simulink model "pid_simulation"  (R2014b)
settings: Solver=ode45  StartTime=0.0  StopTime=20  RelTol=1e-3
values from neighbouring files (symbols this model uses):
  con_D = 0    [main.m]
  con_I = 0    [main.m]
  con_P = 30    [main.m]
  k_velocity_feedback = 3.2    [main.m]
  state_initial = [0 0 0 0 0 0 0 0 0 0 0 0]    [main.m]
libraries: simulink x4
settings Model: Creator=shuoli  LastModifiedBy=shuoli

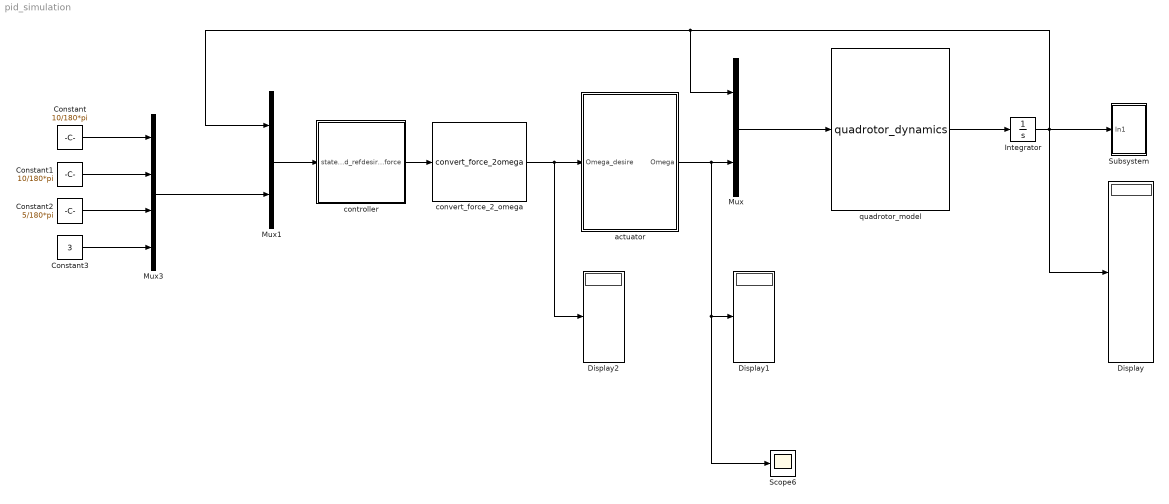
== system pid_simulation ==
  Constant : Constant  Value=10/180*pi
  Constant1 : Constant  Value=10/180*pi
  Constant2 : Constant  Value=5/180*pi
  Constant3 : Constant  Value=3
  Display : Display
  Display1 : Display
  Display2 : Display
  Integrator : Integrator  InitialCondition=state_initial
  Mux : Mux  Inputs=2
  Mux1 : Mux  Inputs=2
  Mux3 : Mux
  Scope6 : Scope
      settings: YMax=2  SaveName=ScopeData17
  Subsystem : Subsystem
  actuator : Subsystem
  controller : Subsystem
  convert_force_2_omega : MATLABFcn  MATLABFcn=convert_force_2omega
  quadrotor_model : MATLABFcn  MATLABFcn=quadrotor_dynamics
  wires:
  quadrotor_model/1 -> Integrator/1
  Mux/1 -> quadrotor_model/1
  Integrator/1 -> Display/1, Mux1/1, Mux/1, Subsystem/1(In1)
  actuator/1(Omega) -> Scope6/1, Display1/1, Mux/2
  Constant3/1 -> Mux3/4
  Constant2/1 -> Mux3/3
  Constant1/1 -> Mux3/2
  Constant/1 -> Mux3/1
  convert_force_2_omega/1 -> Display2/1, actuator/1(Omega_desire)
  Mux3/1 -> Mux1/2
  controller/1(desired_force) -> convert_force_2_omega/1
  Mux1/1 -> controller/1(state_and_ref)

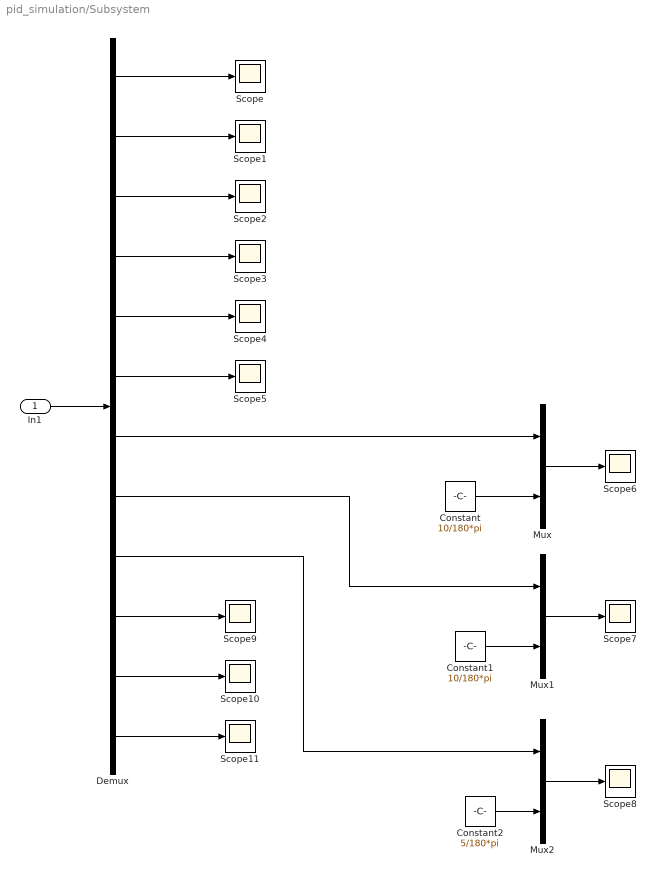
== system pid_simulation/Subsystem ==
  In1 : Inport
  Constant : Constant  Value=10/180*pi
  Constant1 : Constant  Value=10/180*pi
  Constant2 : Constant  Value=5/180*pi
  Demux : Demux  Outputs=12
  Mux : Mux  Inputs=2
  Mux1 : Mux  Inputs=2
  Mux2 : Mux  Inputs=2
  Scope{,1..11} (12 alike) : Scope
      Scope settings: YMin=186  YMax=190
      Scope10 settings: SaveName=ScopeData10
      Scope11 settings: SaveName=ScopeData11
      Scope2 settings: YMin=-18500  YMax=-16500  SaveName=ScopeData2
      Scope3 settings: SaveName=ScopeData3
      Scope4 settings: SaveName=ScopeData4
      Scope5 settings: SaveName=ScopeData5
      Scope6 settings: YMax=2  SaveName=ScopeData6
      Scope7 settings: YMax=2  SaveName=ScopeData7
      Scope8 settings: YMax=2  SaveName=ScopeData8
      Scope9 settings: SaveName=ScopeData9
  wires:
  Demux/1 -> Scope/1
  In1/1 -> Demux/1
  Demux/4 -> Scope3/1
  Demux/2 -> Scope1/1
  Demux/3 -> Scope2/1
  Demux/5 -> Scope4/1
  Demux/6 -> Scope5/1
  Demux/8 -> Mux1/1
  Demux/9 -> Mux2/1
  Demux/10 -> Scope9/1
  Demux/11 -> Scope10/1
  Demux/12 -> Scope11/1
  Demux/7 -> Mux/1
  Mux/1 -> Scope6/1
  Constant/1 -> Mux/2
  Constant1/1 -> Mux1/2
  Mux1/1 -> Scope7/1
  Constant2/1 -> Mux2/2
  Mux2/1 -> Scope8/1

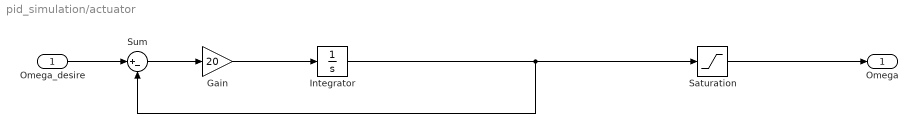
== system pid_simulation/actuator ==
  Omega_desire : Inport
  Gain : Gain  Gain=20
  Integrator : Integrator  InitialCondition=[4477,4477,4477,4477]
  Saturation : Saturate  UpperLimit=8000  LowerLimit=0
  Sum : Sum  Inputs=|+-
  Omega : Outport
  wires:
  Integrator/1 -> Sum/2, Saturation/1
  Omega_desire/1 -> Sum/1
  Sum/1 -> Gain/1
  Gain/1 -> Integrator/1
  Saturation/1 -> Omega/1

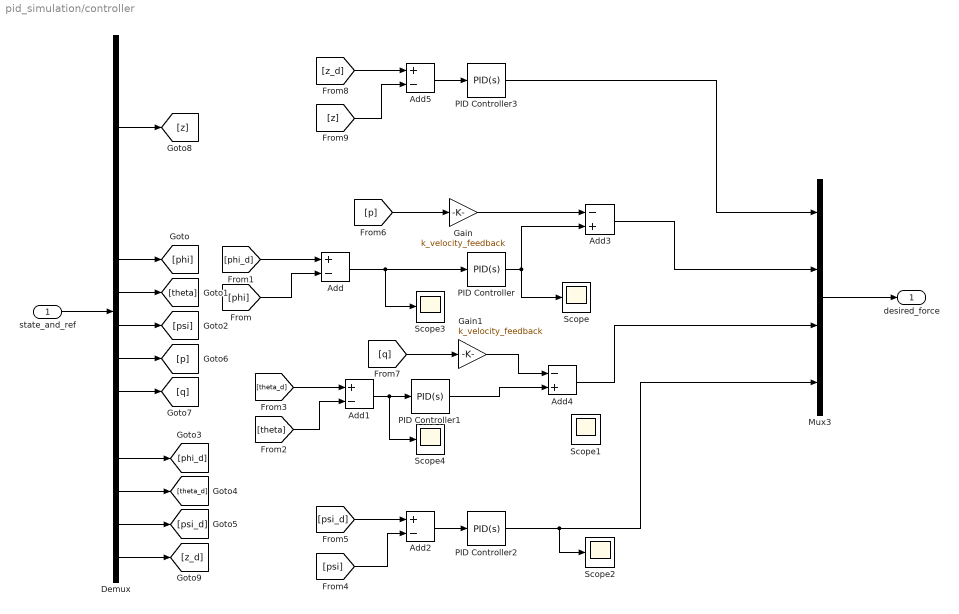
== system pid_simulation/controller ==
  state_and_ref : Inport
  Add{,1..2,5} (4 alike) : Sum  Inputs=+-
  Add3 : Sum  Inputs=-+
  Add4 : Sum  Inputs=-+
  Demux : Demux  Outputs=16
  Gain : Gain  Gain=k_velocity_feedback
  Gain1 : Gain  Gain=k_velocity_feedback
  Mux3 : Mux
  PID Controller : simulink/Continuous/PID Controller  Controller=PID  TimeDomain=Continuous-time  SampleTime=-1  IntegratorMethod=Forward Euler  FilterMethod=Forward Euler  Form=Parallel  P=con_P  I=con_I  D=con_D  N=100  InitialConditionSource=internal  InitialConditionForIntegrator=0  InitialConditionForFilter=0  ExternalReset=none  LimitOutput=off  UpperSaturationLimit=inf  LowerSaturationLimit=-inf  LinearizeAsGain=on  AntiWindupMode=none  Kb=1  TrackingMode=off  Kt=1  PParamMin=[]  PParamMax=[]  IParamMin=[]  IParamMax=[]  DParamMin=[]  DParamMax=[]  NParamMin=[]  NParamMax=[]  KbParamMin=[]  KbParamMax=[]  KtParamMin=[]  KtParamMax=[]  POutMin=[]  POutMax=[]  IOutMin=[]  IOutMax=[]  DOutMin=[]  DOutMax=[]  NOutMin=[]  NOutMax=[]  KbOutMin=[]  KbOutMax=[]  KtOutMin=[]  KtOutMax=[]  IntegratorOutMin=[]  IntegratorOutMax=[]  FilterOutMin=[]  FilterOutMax=[]  SumOutMin=[]  SumOutMax=[]  SumI1OutMin=[]  SumI1OutMax=[]  SumI2OutMin=[]  SumI2OutMax=[]  SumI3OutMin=[]  SumI3OutMax=[]  SumDOutMin=[]  SumDOutMax=[]  SaturationOutMin=[]  SaturationOutMax=[]  IntegratorContinuousStateAttributes=''  IntegratorStateMustResolveToSignalObject=off  IntegratorRTWStateStorageClass=Auto  FilterContinuousStateAttributes=''  FilterStateMustResolveToSignalObject=off  FilterRTWStateStorageClass=Auto  DifferentiatorICPrevScaledInput=0  DifferentiatorOutMin=[]  DifferentiatorOutMax=[]  UseFilter=on
  PID Controller1 : simulink/Continuous/PID Controller  Controller=PID  TimeDomain=Continuous-time  SampleTime=-1  IntegratorMethod=Forward Euler  FilterMethod=Forward Euler  Form=Parallel  P=con_P  I=con_I  D=con_D  N=100  InitialConditionSource=internal  InitialConditionForIntegrator=0  InitialConditionForFilter=0  ExternalReset=none  LimitOutput=off  UpperSaturationLimit=inf  LowerSaturationLimit=-inf  LinearizeAsGain=on  AntiWindupMode=none  Kb=1  TrackingMode=off  Kt=1  PParamMin=[]  PParamMax=[]  IParamMin=[]  IParamMax=[]  DParamMin=[]  DParamMax=[]  NParamMin=[]  NParamMax=[]  KbParamMin=[]  KbParamMax=[]  KtParamMin=[]  KtParamMax=[]  POutMin=[]  POutMax=[]  IOutMin=[]  IOutMax=[]  DOutMin=[]  DOutMax=[]  NOutMin=[]  NOutMax=[]  KbOutMin=[]  KbOutMax=[]  KtOutMin=[]  KtOutMax=[]  IntegratorOutMin=[]  IntegratorOutMax=[]  FilterOutMin=[]  FilterOutMax=[]  SumOutMin=[]  SumOutMax=[]  SumI1OutMin=[]  SumI1OutMax=[]  SumI2OutMin=[]  SumI2OutMax=[]  SumI3OutMin=[]  SumI3OutMax=[]  SumDOutMin=[]  SumDOutMax=[]  SaturationOutMin=[]  SaturationOutMax=[]  IntegratorContinuousStateAttributes=''  IntegratorStateMustResolveToSignalObject=off  IntegratorRTWStateStorageClass=Auto  FilterContinuousStateAttributes=''  FilterStateMustResolveToSignalObject=off  FilterRTWStateStorageClass=Auto  DifferentiatorICPrevScaledInput=0  DifferentiatorOutMin=[]  DifferentiatorOutMax=[]  UseFilter=on
  PID Controller2 : simulink/Continuous/PID Controller  Controller=PID  TimeDomain=Continuous-time  SampleTime=-1  IntegratorMethod=Forward Euler  FilterMethod=Forward Euler  Form=Parallel  P=0.005  I=0  D=0.08  N=100  InitialConditionSource=internal  InitialConditionForIntegrator=0  InitialConditionForFilter=0  ExternalReset=none  LimitOutput=off  UpperSaturationLimit=inf  LowerSaturationLimit=-inf  LinearizeAsGain=on  AntiWindupMode=none  Kb=1  TrackingMode=off  Kt=1  PParamMin=[]  PParamMax=[]  IParamMin=[]  IParamMax=[]  DParamMin=[]  DParamMax=[]  NParamMin=[]  NParamMax=[]  KbParamMin=[]  KbParamMax=[]  KtParamMin=[]  KtParamMax=[]  POutMin=[]  POutMax=[]  IOutMin=[]  IOutMax=[]  DOutMin=[]  DOutMax=[]  NOutMin=[]  NOutMax=[]  KbOutMin=[]  KbOutMax=[]  KtOutMin=[]  KtOutMax=[]  IntegratorOutMin=[]  IntegratorOutMax=[]  FilterOutMin=[]  FilterOutMax=[]  SumOutMin=[]  SumOutMax=[]  SumI1OutMin=[]  SumI1OutMax=[]  SumI2OutMin=[]  SumI2OutMax=[]  SumI3OutMin=[]  SumI3OutMax=[]  SumDOutMin=[]  SumDOutMax=[]  SaturationOutMin=[]  SaturationOutMax=[]  IntegratorContinuousStateAttributes=''  IntegratorStateMustResolveToSignalObject=off  IntegratorRTWStateStorageClass=Auto  FilterContinuousStateAttributes=''  FilterStateMustResolveToSignalObject=off  FilterRTWStateStorageClass=Auto  DifferentiatorICPrevScaledInput=0  DifferentiatorOutMin=[]  DifferentiatorOutMax=[]  UseFilter=on
  PID Controller3 : simulink/Continuous/PID Controller  Controller=PID  TimeDomain=Continuous-time  SampleTime=-1  IntegratorMethod=Forward Euler  FilterMethod=Forward Euler  Form=Parallel  P=20  I=2  D=5  N=100  InitialConditionSource=internal  InitialConditionForIntegrator=0  InitialConditionForFilter=0  ExternalReset=none  LimitOutput=off  UpperSaturationLimit=inf  LowerSaturationLimit=-inf  LinearizeAsGain=on  AntiWindupMode=none  Kb=1  TrackingMode=off  Kt=1  PParamMin=[]  PParamMax=[]  IParamMin=[]  IParamMax=[]  DParamMin=[]  DParamMax=[]  NParamMin=[]  NParamMax=[]  KbParamMin=[]  KbParamMax=[]  KtParamMin=[]  KtParamMax=[]  POutMin=[]  POutMax=[]  IOutMin=[]  IOutMax=[]  DOutMin=[]  DOutMax=[]  NOutMin=[]  NOutMax=[]  KbOutMin=[]  KbOutMax=[]  KtOutMin=[]  KtOutMax=[]  IntegratorOutMin=[]  IntegratorOutMax=[]  FilterOutMin=[]  FilterOutMax=[]  SumOutMin=[]  SumOutMax=[]  SumI1OutMin=[]  SumI1OutMax=[]  SumI2OutMin=[]  SumI2OutMax=[]  SumI3OutMin=[]  SumI3OutMax=[]  SumDOutMin=[]  SumDOutMax=[]  SaturationOutMin=[]  SaturationOutMax=[]  IntegratorContinuousStateAttributes=''  IntegratorStateMustResolveToSignalObject=off  IntegratorRTWStateStorageClass=Auto  FilterContinuousStateAttributes=''  FilterStateMustResolveToSignalObject=off  FilterRTWStateStorageClass=Auto  DifferentiatorICPrevScaledInput=0  DifferentiatorOutMin=[]  DifferentiatorOutMax=[]  UseFilter=on
  Scope{,1..4} (5 alike) : Scope
      Scope settings: YMin=-0.6  YMax=0.4  SaveName=ScopeData12
      Scope1 settings: YMin=-2.6  YMax=-2  SaveName=ScopeData13
      Scope2 settings: YMin=-7450  YMax=-7150  SaveName=ScopeData14
      Scope3 settings: YMin=-3000  YMax=0  SaveName=ScopeData15
      Scope4 settings: SaveName=ScopeData16
  desired_force : Outport
  wires:
  state_and_ref/1 -> Demux/1
  Mux3/1 -> desired_force/1
  PID Controller/1 -> Scope/1, Add3/2
  PID Controller2/1 -> Scope2/1, Mux3/4
  PID Controller3/1 -> Mux3/1
  Demux/13 -> [phi_d]
  Demux/14 -> [theta_d]
  Demux/15 -> [psi_d]
  Add/1 -> Scope3/1, PID Controller/1
  [phi_d] -> Add/1
  [phi] -> Add/2
  Add1/1 -> Scope4/1, PID Controller1/1
  [theta_d] -> Add1/1
  [theta] -> Add1/2
  Add2/1 -> PID Controller2/1
  [psi_d] -> Add2/1
  [psi] -> Add2/2
  Demux/7 -> [phi]
  Demux/8 -> [theta]
  Demux/9 -> [psi]
  Demux/10 -> [p]
  [p] -> Gain/1
  Gain/1 -> Add3/1
  Add3/1 -> Mux3/2
  PID Controller1/1 -> Add4/2
  Add4/1 -> Mux3/3
  Demux/11 -> [q]
  [q] -> Gain1/1
  Gain1/1 -> Add4/1
  Demux/3 -> [z]
  Demux/16 -> [z_d]
  [z_d] -> Add5/1
  [z] -> Add5/2
  Add5/1 -> PID Controller3/1
